simulink model "variable_estado_discreto"  (R2015a)
settings: Solver=ode45  StartTime=0.0  StopTime=100  RelTol=1e-3
values from neighbouring files (symbols this model uses):
  Ad1 = [0.9231]    [variables_estado_disc.m]
  Ad2 = [1.847 -0.8521; 1 0]    [variables_estado_disc.m]
  Ad3 = [0.362 -0.168 0.02556; 1 0 0; 0 1 0]    [variables_estado_disc.m]
  Bd1 = [1]    [variables_estado_disc.m]
  Bd2 = [1;0]    [variables_estado_disc.m]
  Bd3 = [1; 0;0]    [variables_estado_disc.m]
  Cd1 = [0.06727]    [variables_estado_disc.m]
  Cd2 = [0.001847 0.001847]    [variables_estado_disc.m]
  Cd3 = [0.1411 0.2112 0.0224]    [variables_estado_disc.m]
  dend1 = [1 -0.9231]    [variables_estado_disc.m]
  dend2 = [1 -1.847 0.8521]    [variables_estado_disc.m]
  dend3 = [1 -0.362 0.168 -0.02556]    [variables_estado_disc.m]
  numd1 = 0.06727    [variables_estado_disc.m]
  numd2 = [0.001847 0.001847]    [variables_estado_disc.m]
  numd3 = [0.1411 0.2112 0.0224]    [variables_estado_disc.m]
settings Model: CovSFcnEnable=off  Creator=Jose  LastModifiedBy=Administrador
settings DebuggingCC: SolverPrmCheckMsg=warning

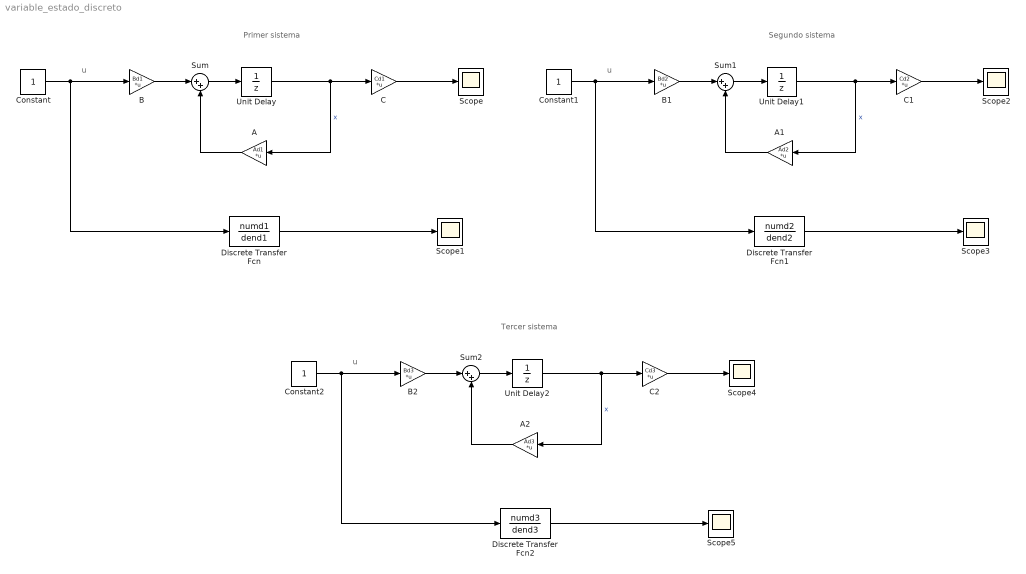
== system variable_estado_discreto ==
  note: Primer sistema
  note: u
  note: Segundo sistema
  note: u
  note: Tercer sistema
  note: u
  A : Gain  Gain=Ad1  Multiplication=Matrix(K*u)  SampleTime=1
  A1 : Gain  Gain=Ad2  Multiplication=Matrix(K*u)  SampleTime=1
  A2 : Gain  Gain=Ad3  Multiplication=Matrix(K*u)  SampleTime=1
  B : Gain  Gain=Bd1  Multiplication=Matrix(K*u)  SampleTime=1
  B1 : Gain  Gain=Bd2  Multiplication=Matrix(K*u)  SampleTime=1
  B2 : Gain  Gain=Bd3  Multiplication=Matrix(K*u)  SampleTime=1
  C : Gain  Gain=Cd1  Multiplication=Matrix(K*u)  SampleTime=1
  C1 : Gain  Gain=Cd2  Multiplication=Matrix(K*u)  SampleTime=1
  C2 : Gain  Gain=Cd3  Multiplication=Matrix(K*u)  SampleTime=1
  Constant : Constant
  Constant1 : Constant
  Constant2 : Constant
  Discrete Transfer Fcn : DiscreteTransferFcn  Numerator=numd1  Denominator=dend1  SampleTime=1
  Discrete Transfer Fcn1 : DiscreteTransferFcn  Numerator=numd2  Denominator=dend2  SampleTime=1
  Discrete Transfer Fcn2 : DiscreteTransferFcn  Numerator=numd3  Denominator=dend3  SampleTime=1
  Scope{,1..5} (6 alike) : Scope
      Scope settings: TimeRange=10
      Scope2 settings: TimeRange=10  SaveName=ScopeData2
      Scope3 settings: SaveName=ScopeData3
      Scope4 settings: TimeRange=10  SaveName=ScopeData4
      Scope5 settings: SaveName=ScopeData5
  Sum : Sum  Inputs=|++
  Sum1 : Sum  Inputs=|++
  Sum2 : Sum  Inputs=|++
  Unit Delay : UnitDelay
  Unit Delay1 : UnitDelay
  Unit Delay2 : UnitDelay
  wires:
  Constant/1 -> Discrete Transfer Fcn/1, B/1
  B/1 -> Sum/1
  Sum/1 -> Unit Delay/1
  Unit Delay/1 -> C/1, A/1  "x"
  A/1 -> Sum/2
  C/1 -> Scope/1
  Discrete Transfer Fcn/1 -> Scope1/1
  Constant1/1 -> Discrete Transfer Fcn1/1, B1/1
  B1/1 -> Sum1/1
  Sum1/1 -> Unit Delay1/1
  Unit Delay1/1 -> C1/1, A1/1  "x"
  A1/1 -> Sum1/2
  C1/1 -> Scope2/1
  Discrete Transfer Fcn1/1 -> Scope3/1
  Constant2/1 -> Discrete Transfer Fcn2/1, B2/1
  B2/1 -> Sum2/1
  Sum2/1 -> Unit Delay2/1
  Unit Delay2/1 -> C2/1, A2/1  "x"
  A2/1 -> Sum2/2
  C2/1 -> Scope4/1
  Discrete Transfer Fcn2/1 -> Scope5/1
